simulink subsystem "Controler_la_force"  (R2020a)
settings: Solver=VariableStepAuto  StartTime=0.0  StopTime=10.0  RelTol=1e-3
model mask{K_c=1.422, K_amp=4.7, L_b=212, R_b=13.75, R_eq=5, B=0.1128, N=66, r=0.0203, V_offset=0.823}
  mask prompts: K_c "Gain du capteur de courant (V/A)"; K_amp "Gain de l'amplificateur"; L_b "Inductance de la bobine (uH)"; R_b "Résistance de la bobine (ohm)"; R_eq "Résistance équivalente de l'amplificateur"; B "Magnitude du champ d'induction magnétique (Tesla)"; N "Nombre de tours de la bobine"; r "Rayon de la bobine (m)"; V_offset "Voltage de l'offset"
values from neighbouring files (symbols this model uses):
  K_amp = 4.7    [default_design_data.mat]    (also in dict.sldd)
  K_c = 1.422    [default_design_data.mat]    (also in dict.sldd)
  R_eq = 1.1    [default_design_data.mat]
libraries: simulink x1
settings Model: Creator=frfoc1  LastModifiedBy=MAGUY18

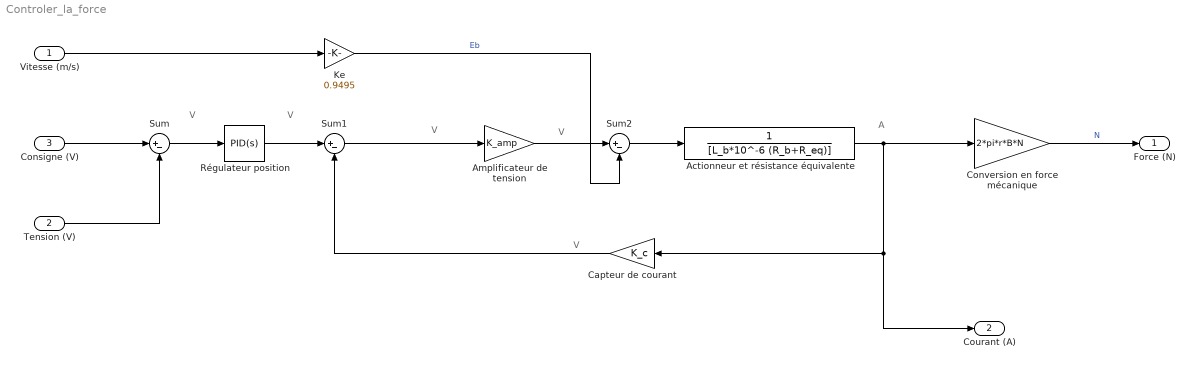
== system Controler_la_force ==
  note: A
  note: V
  note: V
  note: V
  note: V
  note: V
  Vitesse (m/s) : Inport
  Tension (V) : Inport  Port=2
  Consigne (V) : Inport  Port=3
  Actionneur et résistance équivalente : TransferFcn  Denominator=[L_b*10^-6 (R_b+R_eq)]
  Amplificateur de tension : Gain  Gain=K_amp
  Capteur de courant : Gain  Gain=K_c
  Conversion en force mécanique : Gain  Gain=2*pi*r*B*N
  Ke : Gain  Gain=0.9495
  Régulateur position : simulink/Continuous/PID Controller  Controller=PID  Form=Parallel  TimeDomain=Continuous-time  UseExternalTs=off  SampleTime=-1  IntegratorMethod=Forward Euler  FilterMethod=Forward Euler  ControllerParametersSource=internal  P=112.5  I=1125  D=0  UseFilter=on  N=100  TunerSelectOption=Transfer Function Based (PID Tuner App)  InitialConditionSource=internal  InitialConditionForIntegrator=0  InitialConditionForFilter=0  DifferentiatorICPrevScaledInput=0  ExternalReset=none  TrackingMode=off  Kt=1  LimitOutput=off  UpperSaturationLimit=inf  LowerSaturationLimit=-inf  LinearizeAsGain=on  AntiWindupMode=none  Kb=1  POutMin=[]  POutMax=[]  IOutMin=[]  IOutMax=[]  DOutMin=[]  DOutMax=[]  NOutMin=[]  NOutMax=[]  SumOutMin=[]  SumOutMax=[]  SaturationOutMin=[]  SaturationOutMax=[]  PParamMin=[]  PParamMax=[]  IParamMin=[]  IParamMax=[]  DParamMin=[]  DParamMax=[]  NParamMin=[]  NParamMax=[]  KbParamMin=[]  KbParamMax=[]  KtParamMin=[]  KtParamMax=[]  KbOutMin=[]  KbOutMax=[]  KtOutMin=[]  KtOutMax=[]  IntegratorOutMin=[]  IntegratorOutMax=[]  FilterOutMin=[]  FilterOutMax=[]  SumI1OutMin=[]  SumI1OutMax=[]  SumI2OutMin=[]  SumI2OutMax=[]  SumI3OutMin=[]  SumI3OutMax=[]  SumI4OutMin=[]  SumI4OutMax=[]  SumDOutMin=[]  SumDOutMax=[]  DifferentiatorOutMin=[]  DifferentiatorOutMax=[]  FilterDiffOutCoefMin=[]  FilterDiffOutCoefMax=[]  ReciprocalOutMin=[]  ReciprocalOutMax=[]  SumDenOutMin=[]  SumDenOutMax=[]  SumNumOutMin=[]  SumNumOutMax=[]  DivideOutMin=[]  DivideOutMax=[]  UdiffTsProdOutMin=[]  UdiffTsProdOutMax=[]  NTsProdOutMin=[]  NTsProdOutMax=[]  UintegralTsProdOutMin=[]  UintegralTsProdOutMax=[]  UngainTsProdOutMin=[]  UngainTsProdOutMax=[]  IntegratorContinuousStateAttributes=''  IntegratorStateMustResolveToSignalObject=off  IntegratorRTWStateStorageClass=Auto  FilterContinuousStateAttributes=''  FilterStateMustResolveToSignalObject=off  FilterRTWStateStorageClass=Auto  ParallelPVariant=InternalParameters  IdealPVariant=Disabled  IVariant=InternalParameters  DVariant=InternalParameters  IntegratorVariant=Continuous  SatVariant=Disabled  AWVariant=Passthrough  PCopyVariant=Disabled  TRVariant=Disabled  FdbkBlocksVariant=Forward  IdealPFdbkVariant=Disabled  SatFdbkVariant=Disabled  DerivativeFilterVariant=ContFilter  NVariant=InternalParameters  NCopyVariant=Disabled  FilterICVariant=InternalICsFilter  IntegratorICVariant=InternalICs  ExternalResetVariant=Disabled  TRSumVariant=Passthrough  SumFdbkVariant=Disabled  SumVariant=Sum_PID  TsampFilterVariant=InternalTs  TsampNgainVariant=Passthrough  TsampIntegralVariant=Passthrough
  Sum : Sum  Inputs=|+-
  Sum1 : Sum  Inputs=|+-
  Sum2 : Sum  Inputs=|+-
  Force (N) : Outport
  Courant (A) : Outport  Port=2
  wires:
  Tension (V)/1 -> Sum/2
  Actionneur et résistance équivalente/1 -> Capteur de courant/1, Courant (A)/1, Conversion en force mécanique/1
  Conversion en force mécanique/1 -> Force (N)/1  "N"
  Capteur de courant/1 -> Sum1/2
  Sum1/1 -> Amplificateur de tension/1
  Sum/1 -> Régulateur position/1
  Régulateur position/1 -> Sum1/1
  Consigne (V)/1 -> Sum/1
  Vitesse (m/s)/1 -> Ke/1
  Amplificateur de tension/1 -> Sum2/1
  Ke/1 -> Sum2/2  "Eb"
  Sum2/1 -> Actionneur et résistance équivalente/1
